simulink model "model1"  (R2024b)
settings: Solver=VariableStepAuto  StartTime=0.0  StopTime=100  RelTol=1e-3
settings Model: Creator=mehmetcanevi  LastModifiedBy=mehmetcanevi

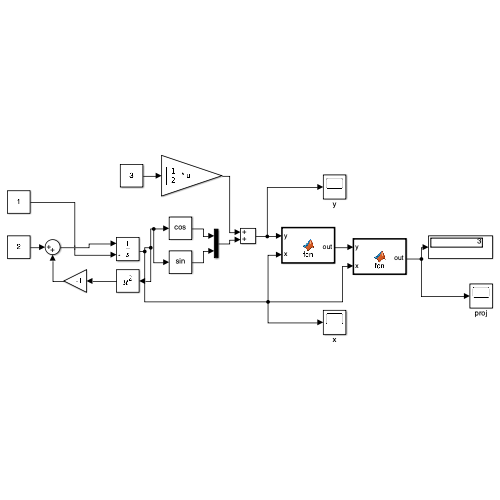
[thumbnail: Simulink's stored preview of the top-level diagram]
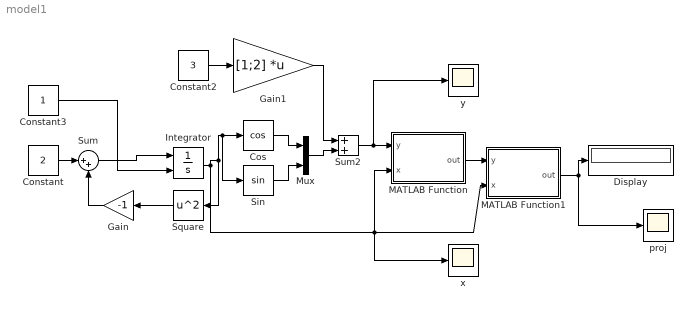
== system model1 ==
  Constant : Constant  Value=2
  Constant2 : Constant  Value=3
  Constant3 : Constant
  Cos : Trigonometry  Operator=cos
  Display : Display
  Gain : Gain  Gain=-1
  Gain1 : Gain  Gain=[1;2]  Multiplication=Matrix(K*u)
  Integrator : Integrator  InitialConditionSource=external
  MATLAB Function : MATLAB Function  TreatAsAtomicUnit=on
  MATLAB Function1 : MATLAB Function  TreatAsAtomicUnit=on
  Mux : Mux  Inputs=2
  Sin : Trigonometry
  Square : Math  Operator=square
  Sum : Sum  Inputs=|++
  Sum2 : Sum
  proj : Scope
  x : Scope
  y : Scope
  wires:
  Integrator/1 -> Square/1, Sin/1, Cos/1, MATLAB Function/2(x), MATLAB Function1/2(x), x/1
  Constant/1 -> Sum/1
  Sum/1 -> Integrator/1
  Cos/1 -> Mux/1
  MATLAB Function1/1(out) -> Display/1, proj/1
  Square/1 -> Gain/1
  Gain/1 -> Sum/2
  Constant3/1 -> Integrator/2
  Sin/1 -> Mux/2
  Mux/1 -> Sum2/2
  Constant2/1 -> Gain1/1
  Gain1/1 -> Sum2/1
  Sum2/1 -> y/1, MATLAB Function/1(y)
  MATLAB Function/1(out) -> MATLAB Function1/1(y)

== matlab function model1/MATLAB Function ==
  data: y input; out output; x input
function out= fcn(y,x)
out=[sin(x)^2, -sin(x)*cos(x);-sin(x)*cos(x), cos(x)^2]*y;
end

== matlab function model1/MATLAB Function1 ==
  data: y input; out output; x input
function out= fcn(y,x)
out=[-(sin(2*x) + cos(x)^2 - 1)/(3*cos(x)^2 - 2*sin(2*x) + 1), (cos(x)*(2*cos(x) - sin(x)))/(3*cos(x)^2 - 2*sin(2*x) + 1)]*y;
end
